simulink model "ObserverJacobian"  (R2022b)
settings: Solver=FixedStepAuto  StartTime=0.0  StopTime=10.0  RelTol=1e-3  SampleTimeConstraint=STIndependent
undefined symbols (not defined in the file): NumberSt, NumModules, NumSeries
settings Model: DataDictionary=Estimators_Dictionary.sldd  Creator=japerez  LastModifiedBy=jgavidia
settings DataIOCC: SaveOutput=off  SaveTime=off
settings DebuggingCC: ParameterPrecisionLossMsg=none

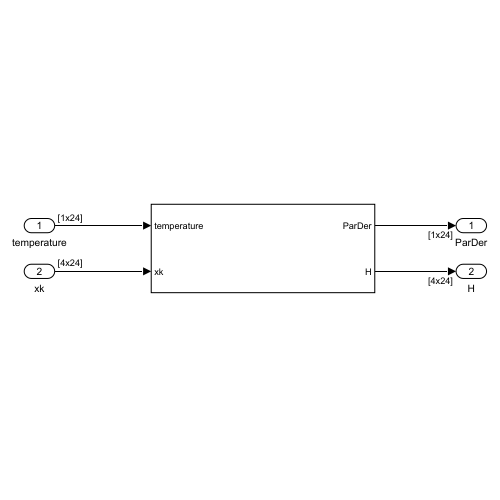
[thumbnail: Simulink's stored preview of the top-level diagram]
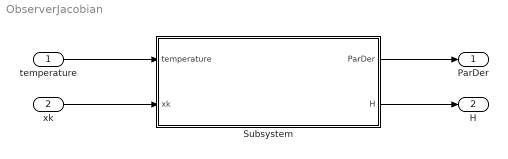
== system ObserverJacobian ==
  temperature : Inport  OutDataTypeStr=single  PortDimensions=[1,NumModules*NumSeries]
  xk : Inport  Port=2  OutDataTypeStr=single  PortDimensions=[NumberSt,NumModules*NumSeries]
  Subsystem : Subsystem
  ParDer : Outport  OutDataTypeStr=single  PortDimensions=[1,NumModules*NumSeries]
  H : Outport  Port=2  OutDataTypeStr=single  PortDimensions=[NumberSt,NumModules*NumSeries]
  wires:
  xk/1 -> Subsystem/2(xk)
  Subsystem/1(ParDer) -> ParDer/1
  temperature/1 -> Subsystem/1(temperature)
  Subsystem/2(H) -> H/1

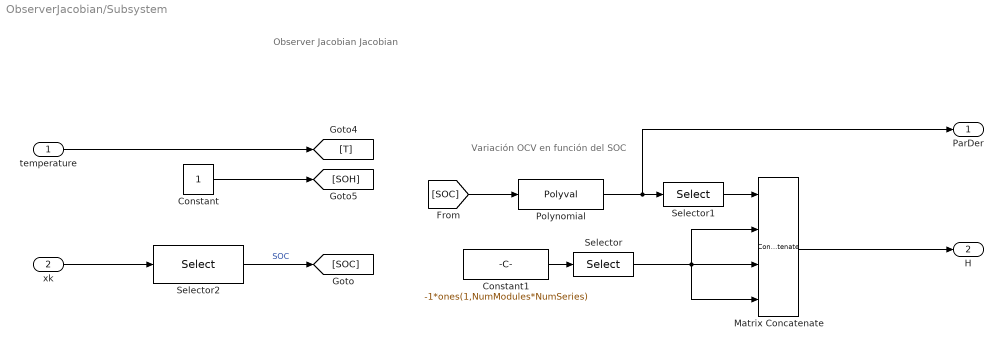
== system ObserverJacobian/Subsystem ==
  note: Observer Jacobian Jacobian
  note: Variación OCV en función del SOC
  temperature : Inport
  xk : Inport  Port=2
  Constant : Constant
  Constant1 : Constant  Value=-1*ones(1,NumModules*NumSeries)  OutDataTypeStr=single
  Matrix Concatenate : Concatenate  NumInputs=4  Mode=Multidimensional array
  Polynomial : Polyval  Coefs=[-7.321*4,17.55*3,-14.72*2,5.972]
  Selector : Selector  NumberOfDimensions=2  InputPortWidth=3  IndexOptions=Select all,Index vector (dialog)  Indices=[1 3],[1:24]  OutputSizes=1,1
  Selector1 : Selector  NumberOfDimensions=2  InputPortWidth=3  IndexOptions=Select all,Index vector (dialog)  Indices=[1 3],[1:24]  OutputSizes=1,1
  Selector2 : Selector  NumberOfDimensions=2  InputPortWidth=24  IndexOptions=Index vector (dialog),Select all  Indices=1,1  OutputSizes=1,1
  ParDer : Outport
  H : Outport  Port=2
  wires:
  xk/1 -> Selector2/1
  temperature/1 -> [T]
  [SOC] -> Polynomial/1
  Polynomial/1 -> Selector1/1, ParDer/1
  Selector2/1 -> [SOC]  "SOC"
  Constant/1 -> [SOH]
  Matrix Concatenate/1 -> H/1
  Constant1/1 -> Selector/1
  Selector/1 -> Matrix Concatenate/4, Matrix Concatenate/3, Matrix Concatenate/2
  Selector1/1 -> Matrix Concatenate/1
